simulink model "ConsolidatedModelV3"  (R2022a)
settings: Solver=VariableStepAuto  StartTime=0.0  StopTime=10.0  RelTol=1e-3
undefined symbols (not defined in the file or in its folder): s0
libraries: rllib x1
settings Model: Creator=yangz  LastModifiedBy=yangz

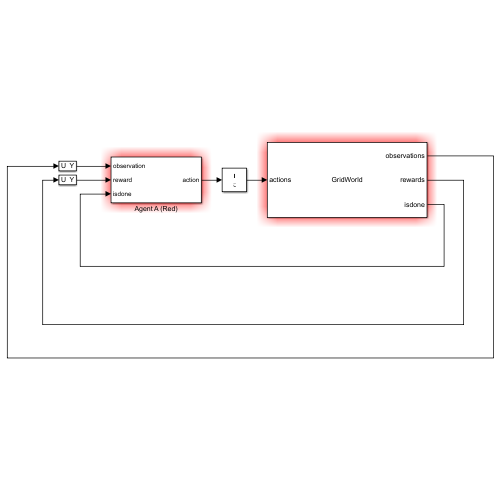
[thumbnail: Simulink's stored preview of the top-level diagram]
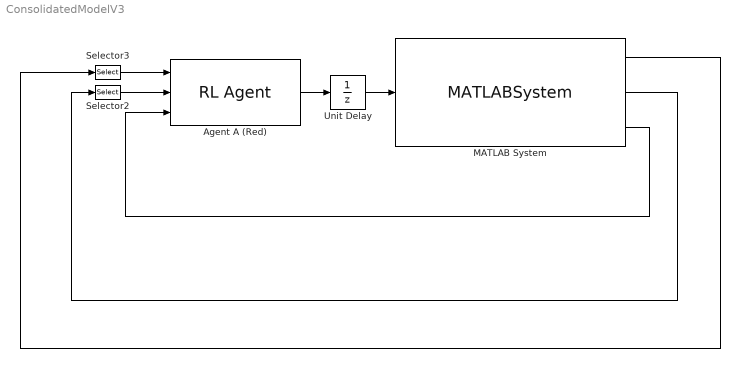
== system ConsolidatedModelV3 ==
  Agent A (Red) : rllib/RL Agent  Agent=agent1  ExternalActionAsInput=off  ProvideLastAction=off  ProvideCumRwd=off  TreatAsDirectFeedthrough=on  UseStrictObservationDataTypes=off
  MATLAB System : MATLABSystem  System=GridWorld  InitialStates=s0  Obstacles=obsMat  MaxStepCount=maxsteps  SimulateUsing=Interpreted execution
      mask Type: GridWorld
      mask Display:
      | disp('GridWorld');
      | port_label('input',1,'actions');
      | port_label('output',1,'observations');
      | port_label('output',2,'rewards');
      | port_label('output',3,'isdone');
  Selector2 : Selector  InputPortWidth=3  IndexOptions=Index vector (dialog)  Indices=1  OutputSizes=1
  Selector3 : Selector  NumberOfDimensions=4  InputPortWidth=3  IndexOptions=Select all,Select all,Select all,Index vector (dialog)  Indices=1,1,1,1  OutputSizes=1,1,1,1
  Unit Delay : UnitDelay  SampleTime=-1  HasFrameUpgradeWarning=on
  wires:
  Agent A (Red)/1 -> Unit Delay/1
  Unit Delay/1 -> MATLAB System/1
  Selector3/1 -> Agent A (Red)/1
  Selector2/1 -> Agent A (Red)/2
  MATLAB System/1 -> Selector3/1
  MATLAB System/2 -> Selector2/1
  MATLAB System/3 -> Agent A (Red)/3
